simulink model "p1_digital_twin_R2023a"  (R2023a)
settings: Solver=FixedStepDiscrete  StartTime=0.0  StopTime=10  FixedStep=Ts  RelTol=1e-3  EnableMultiTasking=on
values from neighbouring files (symbols this model uses):
  ack = 1    [SteeringController.m]
  cpr_handwheel = 500*4    (= 2000)    [p1_params_new.m]
  cpr_steering = 1000*4    (= 4000)    [p1_params_new.m]
  hal_filter_den = [1 1*(2*pi*Ts)-1]    [SteeringController.m]    (also in p1_params_new.m = DEN_cellarray{1})
  hal_filter_num = [1*(2*pi*Ts)]    [SteeringController.m]    (also in p1_params_new.m = NUM_cellarray{1})
  n_drive = 5.6    [p1_params_new.m]
  n_handwheel = 50    [p1_params_new.m]
  n_steering = 160    [p1_params_new.m]
  sr = 7.5    [SteeringController.m]
  steering_limit = 35    [SteeringController.m]
  Ts = 0.001    [p1_params_new.m]
  wc = 10    [SteeringController.m]    (also in p1_params_new.m = p1params.input.VAccelFc*(2*Ts))
undefined symbols (not defined in the file or in its folder): DiscIntNeverNeededParam, p1params, param
libraries: simulink x7
(part 2 of 4)

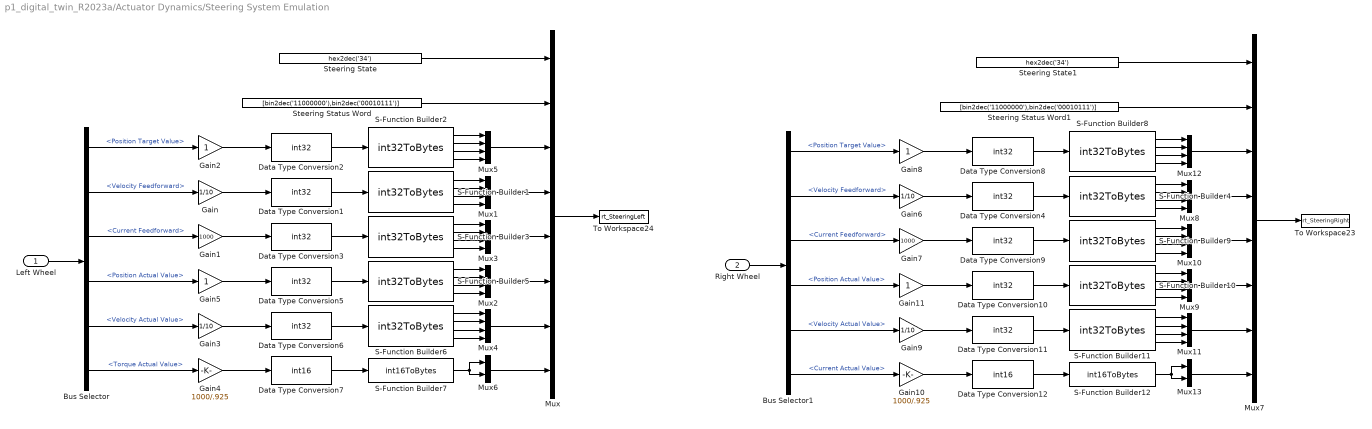
== system p1_digital_twin_R2023a/Actuator Dynamics/Steering System Emulation ==
  Left Wheel : Inport
  Right Wheel : Inport  Port=2
  Bus Selector : BusSelector  OutputSignals=Position Target Value,Velocity Feedforward,Current Feedforward,Position Actual Value,Velocity Actual Value,Torque Actual Value
  Bus Selector1 : BusSelector  OutputSignals=Position Target Value,Velocity Feedforward,Current Feedforward,Position Actual Value,Velocity Actual Value,Current Actual Value
  Data Type Conversion{1..6,8..11} (10 alike) : DataTypeConversion  OutDataTypeStr=int32  RndMeth=Floor
  Data Type Conversion12 : DataTypeConversion  OutDataTypeStr=int16  RndMeth=Floor
  Data Type Conversion7 : DataTypeConversion  OutDataTypeStr=int16  RndMeth=Floor
  Gain{,3,6,9} (4 alike) : Gain  Gain=1/10
  Gain1 : Gain  Gain=1000
  Gain10 : Gain  Gain=1000/.925
  Gain{2,5,8,11} (4 alike) : Gain
  Gain4 : Gain  Gain=1000/.925
  Gain7 : Gain  Gain=1000
  Mux : Mux  Inputs=8
  Mux{1..5,8..12} (10 alike) : Mux
  Mux13 : Mux  Inputs=2
  Mux6 : Mux  Inputs=2
  Mux7 : Mux  Inputs=8
  S-Function Builder1 : S-Function  FunctionName=int32ToBytes  SFunctionModules=int32ToBytes_wrapper.c  SFunctionDeploymentMode=off  EnableBusSupport=off  mask(S-Function Builder){}
      mask help: Simulink:masks:SFunctionBuilder_MD
      mask init:
      | val = [[.9  0.75 0.75 1 1 .9 .9 1]',[1 1 0.75 0.75 .9 .9 1 .9]'];try , sys = get_param(gcb,'SfunBuilderFcnName');if isempty(sys), sys = get_param(gcb,'FunctionName'); end,catch, sys = get_param(gcb,'FunctionName'); end
      settings: CopyFcn=set_param(gcbh,'LinkStatus','none')  OpenFcn=sfunctionwizard(gcbh)
      mask Display:
      | plot(val(:,1),val(:,2))
      | disp(sys)
      | port_label('input',1,'u0')
      | port_label('output',1,'y0')
      | port_label('output',2,'y1')
      | port_label('output',3,'y2')
      | port_label('output',4,'y3')
  S-Function Builder10 : S-Function  FunctionName=int32ToBytes  SFunctionModules=int32ToBytes_wrapper.c  SFunctionDeploymentMode=off  EnableBusSupport=off  mask(S-Function Builder){}
      mask help: Simulink:masks:SFunctionBuilder_MD
      mask init: same as p1_digital_twin_R2023a/Actuator Dynamics/Steering System Emulation/S-Function Builder1
      settings: CopyFcn=set_param(gcbh,'LinkStatus','none')  OpenFcn=sfunctionwizard(gcbh)
      mask Display:
      | plot(val(:,1),val(:,2))
      | disp(sys)
      | port_label('input',1,'u0')
      | port_label('output',1,'y0')
      | port_label('output',2,'y1')
      | port_label('output',3,'y2')
      | port_label('output',4,'y3')
  S-Function Builder11 : S-Function  FunctionName=int32ToBytes  SFunctionModules=int32ToBytes_wrapper.c  SFunctionDeploymentMode=off  EnableBusSupport=off  mask(S-Function Builder){}
      mask help: Simulink:masks:SFunctionBuilder_MD
      mask init: same as p1_digital_twin_R2023a/Actuator Dynamics/Steering System Emulation/S-Function Builder1
      settings: CopyFcn=set_param(gcbh,'LinkStatus','none')  OpenFcn=sfunctionwizard(gcbh)
      mask Display:
      | plot(val(:,1),val(:,2))
      | disp(sys)
      | port_label('input',1,'u0')
      | port_label('output',1,'y0')
      | port_label('output',2,'y1')
      | port_label('output',3,'y2')
      | port_label('output',4,'y3')
  S-Function Builder12 : S-Function  FunctionName=int16ToBytes  SFunctionModules=int16ToBytes_wrapper.c  SFunctionDeploymentMode=off  EnableBusSupport=off  mask(S-Function Builder){}
      mask help: Simulink:masks:SFunctionBuilder_MD
      mask init: same as p1_digital_twin_R2023a/Actuator Dynamics/Steering System Emulation/S-Function Builder1
      settings: CopyFcn=set_param(gcbh,'LinkStatus','none')  OpenFcn=sfunctionwizard(gcbh)
      mask Display:
      | plot(val(:,1),val(:,2))
      | disp(sys)
      | port_label('input',1,'u0')
      | port_label('output',1,'y0')
  S-Function Builder2 : S-Function  FunctionName=int32ToBytes  SFunctionModules=int32ToBytes_wrapper.c  SFunctionDeploymentMode=off  EnableBusSupport=off  mask(S-Function Builder){}
      mask help: Simulink:masks:SFunctionBuilder_MD
      mask init: same as p1_digital_twin_R2023a/Actuator Dynamics/Steering System Emulation/S-Function Builder1
      settings: CopyFcn=set_param(gcbh,'LinkStatus','none')  OpenFcn=sfunctionwizard(gcbh)
      mask Display:
      | plot(val(:,1),val(:,2))
      | disp(sys)
      | port_label('input',1,'u0')
      | port_label('output',1,'y0')
      | port_label('output',2,'y1')
      | port_label('output',3,'y2')
      | port_label('output',4,'y3')
  S-Function Builder3 : S-Function  FunctionName=int32ToBytes  SFunctionModules=int32ToBytes_wrapper.c  SFunctionDeploymentMode=off  EnableBusSupport=off  mask(S-Function Builder){}
      mask help: Simulink:masks:SFunctionBuilder_MD
      mask init: same as p1_digital_twin_R2023a/Actuator Dynamics/Steering System Emulation/S-Function Builder1
      settings: CopyFcn=set_param(gcbh,'LinkStatus','none')  OpenFcn=sfunctionwizard(gcbh)
      mask Display:
      | plot(val(:,1),val(:,2))
      | disp(sys)
      | port_label('input',1,'u0')
      | port_label('output',1,'y0')
      | port_label('output',2,'y1')
      | port_label('output',3,'y2')
      | port_label('output',4,'y3')
  S-Function Builder4 : S-Function  FunctionName=int32ToBytes  SFunctionModules=int32ToBytes_wrapper.c  SFunctionDeploymentMode=off  EnableBusSupport=off  mask(S-Function Builder){}
      mask help: Simulink:masks:SFunctionBuilder_MD
      mask init: same as p1_digital_twin_R2023a/Actuator Dynamics/Steering System Emulation/S-Function Builder1
      settings: CopyFcn=set_param(gcbh,'LinkStatus','none')  OpenFcn=sfunctionwizard(gcbh)
      mask Display:
      | plot(val(:,1),val(:,2))
      | disp(sys)
      | port_label('input',1,'u0')
      | port_label('output',1,'y0')
      | port_label('output',2,'y1')
      | port_label('output',3,'y2')
      | port_label('output',4,'y3')
  S-Function Builder5 : S-Function  FunctionName=int32ToBytes  SFunctionModules=int32ToBytes_wrapper.c  SFunctionDeploymentMode=off  EnableBusSupport=off  mask(S-Function Builder){}
      mask help: Simulink:masks:SFunctionBuilder_MD
      mask init: same as p1_digital_twin_R2023a/Actuator Dynamics/Steering System Emulation/S-Function Builder1
      settings: CopyFcn=set_param(gcbh,'LinkStatus','none')  OpenFcn=sfunctionwizard(gcbh)
      mask Display:
      | plot(val(:,1),val(:,2))
      | disp(sys)
      | port_label('input',1,'u0')
      | port_label('output',1,'y0')
      | port_label('output',2,'y1')
      | port_label('output',3,'y2')
      | port_label('output',4,'y3')
  S-Function Builder6 : S-Function  FunctionName=int32ToBytes  SFunctionModules=int32ToBytes_wrapper.c  SFunctionDeploymentMode=off  EnableBusSupport=off  mask(S-Function Builder){}
      mask help: Simulink:masks:SFunctionBuilder_MD
      mask init: same as p1_digital_twin_R2023a/Actuator Dynamics/Steering System Emulation/S-Function Builder1
      settings: CopyFcn=set_param(gcbh,'LinkStatus','none')  OpenFcn=sfunctionwizard(gcbh)
      mask Display:
      | plot(val(:,1),val(:,2))
      | disp(sys)
      | port_label('input',1,'u0')
      | port_label('output',1,'y0')
      | port_label('output',2,'y1')
      | port_label('output',3,'y2')
      | port_label('output',4,'y3')
  S-Function Builder7 : S-Function  FunctionName=int16ToBytes  SFunctionModules=int16ToBytes_wrapper.c  SFunctionDeploymentMode=off  EnableBusSupport=off  mask(S-Function Builder){}
      mask help: Simulink:masks:SFunctionBuilder_MD
      mask init: same as p1_digital_twin_R2023a/Actuator Dynamics/Steering System Emulation/S-Function Builder1
      settings: CopyFcn=set_param(gcbh,'LinkStatus','none')  OpenFcn=sfunctionwizard(gcbh)
      mask Display:
      | plot(val(:,1),val(:,2))
      | disp(sys)
      | port_label('input',1,'u0')
      | port_label('output',1,'y0')
  S-Function Builder8 : S-Function  FunctionName=int32ToBytes  SFunctionModules=int32ToBytes_wrapper.c  SFunctionDeploymentMode=off  EnableBusSupport=off  mask(S-Function Builder){}
      mask help: Simulink:masks:SFunctionBuilder_MD
      mask init: same as p1_digital_twin_R2023a/Actuator Dynamics/Steering System Emulation/S-Function Builder1
      settings: CopyFcn=set_param(gcbh,'LinkStatus','none')  OpenFcn=sfunctionwizard(gcbh)
      mask Display:
      | plot(val(:,1),val(:,2))
      | disp(sys)
      | port_label('input',1,'u0')
      | port_label('output',1,'y0')
      | port_label('output',2,'y1')
      | port_label('output',3,'y2')
      | port_label('output',4,'y3')
  S-Function Builder9 : S-Function  FunctionName=int32ToBytes  SFunctionModules=int32ToBytes_wrapper.c  SFunctionDeploymentMode=off  EnableBusSupport=off  mask(S-Function Builder){}
      mask help: Simulink:masks:SFunctionBuilder_MD
      mask init: same as p1_digital_twin_R2023a/Actuator Dynamics/Steering System Emulation/S-Function Builder1
      settings: CopyFcn=set_param(gcbh,'LinkStatus','none')  OpenFcn=sfunctionwizard(gcbh)
      mask Display:
      | plot(val(:,1),val(:,2))
      | disp(sys)
      | port_label('input',1,'u0')
      | port_label('output',1,'y0')
      | port_label('output',2,'y1')
      | port_label('output',3,'y2')
      | port_label('output',4,'y3')
  Steering State : Constant  Value=hex2dec('34')  OutDataTypeStr=uint8  SampleTime=-1
  Steering State1 : Constant  Value=hex2dec('34')  OutDataTypeStr=uint8  SampleTime=-1
  Steering Status Word : Constant  Value=[bin2dec('11000000'),bin2dec('00010111')]  OutDataTypeStr=uint8  SampleTime=-1
  Steering Status Word1 : Constant  Value=[bin2dec('11000000'),bin2dec('00010111')]  OutDataTypeStr=uint8  SampleTime=-1
  To Workspace23 : ToWorkspace  VariableName=rt_SteeringRight  SampleTime=-1
  To Workspace24 : ToWorkspace  VariableName=rt_SteeringLeft  SampleTime=-1
  wires:
  Mux/1 -> To Workspace24/1
  Steering State/1 -> Mux/1
  Mux5/1 -> Mux/3
  S-Function Builder2/3 -> Mux5/3
  S-Function Builder2/1 -> Mux5/1
  S-Function Builder2/4 -> Mux5/4
  S-Function Builder2/2 -> Mux5/2
  Steering Status Word/1 -> Mux/2
  S-Function Builder1/4 -> Mux1/4
  S-Function Builder1/1 -> Mux1/1
  S-Function Builder1/2 -> Mux1/2
  S-Function Builder1/3 -> Mux1/3
  Mux1/1 -> Mux/4
  Mux2/1 -> Mux/6
  S-Function Builder3/4 -> Mux3/4
  S-Function Builder3/1 -> Mux3/1
  S-Function Builder3/2 -> Mux3/2
  S-Function Builder3/3 -> Mux3/3
  Mux3/1 -> Mux/5
  S-Function Builder5/3 -> Mux2/3
  S-Function Builder5/1 -> Mux2/1
  S-Function Builder5/2 -> Mux2/2
  S-Function Builder5/4 -> Mux2/4
  Mux4/1 -> Mux/7
  S-Function Builder6/3 -> Mux4/3
  S-Function Builder6/4 -> Mux4/4
  S-Function Builder6/2 -> Mux4/2
  S-Function Builder6/1 -> Mux4/1
  Mux6/1 -> Mux/8
  Data Type Conversion2/1 -> S-Function Builder2/1
  Data Type Conversion1/1 -> S-Function Builder1/1
  Data Type Conversion3/1 -> S-Function Builder3/1
  Data Type Conversion5/1 -> S-Function Builder5/1
  Data Type Conversion6/1 -> S-Function Builder6/1
  Data Type Conversion7/1 -> S-Function Builder7/1
  S-Function Builder7/1 -> Mux6/2, Mux6/1
  Gain2/1 -> Data Type Conversion2/1
  Gain/1 -> Data Type Conversion1/1
  Gain1/1 -> Data Type Conversion3/1
  Gain5/1 -> Data Type Conversion5/1
  Gain3/1 -> Data Type Conversion6/1
  Left Wheel/1 -> Bus Selector/1
  Bus Selector/1 -> Gain2/1  "<Position Target Value>"
  Bus Selector/2 -> Gain/1  "<Velocity Feedforward>"
  Bus Selector/3 -> Gain1/1  "<Current Feedforward>"
  Bus Selector/4 -> Gain5/1  "<Position Actual Value>"
  Bus Selector/5 -> Gain3/1  "<Velocity Actual Value>"
  Bus Selector/6 -> Gain4/1  "<Torque Actual Value>"
  Mux10/1 -> Mux7/5
  Gain9/1 -> Data Type Conversion11/1
  Gain10/1 -> Data Type Conversion12/1
  Right Wheel/1 -> Bus Selector1/1
  S-Function Builder12/1 -> Mux13/2, Mux13/1
  Data Type Conversion11/1 -> S-Function Builder11/1
  Bus Selector1/6 -> Gain10/1  "<Current Actual Value>"
  Mux9/1 -> Mux7/6
  Bus Selector1/3 -> Gain7/1  "<Current Feedforward>"
  Data Type Conversion9/1 -> S-Function Builder9/1
  S-Function Builder9/4 -> Mux10/4
  Gain11/1 -> Data Type Conversion10/1
  S-Function Builder9/3 -> Mux10/3
  S-Function Builder10/4 -> Mux9/4
  Mux12/1 -> Mux7/3
  S-Function Builder11/2 -> Mux11/2
  Data Type Conversion8/1 -> S-Function Builder8/1
  S-Function Builder8/4 -> Mux12/4
  S-Function Builder9/1 -> Mux10/1
  S-Function Builder10/1 -> Mux9/1
  S-Function Builder10/2 -> Mux9/2
  Data Type Conversion10/1 -> S-Function Builder10/1
  Data Type Conversion4/1 -> S-Function Builder4/1
  S-Function Builder4/1 -> Mux8/1
  S-Function Builder8/3 -> Mux12/3
  Mux8/1 -> Mux7/4
  S-Function Builder9/2 -> Mux10/2
  Gain8/1 -> Data Type Conversion8/1
  S-Function Builder8/1 -> Mux12/1
  S-Function Builder8/2 -> Mux12/2
  Steering Status Word1/1 -> Mux7/2
  Steering State1/1 -> Mux7/1
  S-Function Builder11/1 -> Mux11/1
  Gain7/1 -> Data Type Conversion9/1
  S-Function Builder10/3 -> Mux9/3
  Bus Selector1/5 -> Gain9/1  "<Velocity Actual Value>"
  S-Function Builder4/3 -> Mux8/3
  Bus Selector1/1 -> Gain8/1  "<Position Target Value>"
  Bus Selector1/4 -> Gain11/1  "<Position Actual Value>"
  Gain6/1 -> Data Type Conversion4/1
  S-Function Builder4/2 -> Mux8/2
  Bus Selector1/2 -> Gain6/1  "<Velocity Feedforward>"
  S-Function Builder4/4 -> Mux8/4
  Mux11/1 -> Mux7/7
  Mux13/1 -> Mux7/8
  Data Type Conversion12/1 -> S-Function Builder12/1
  S-Function Builder11/4 -> Mux11/4
  S-Function Builder11/3 -> Mux11/3
  Mux7/1 -> To Workspace23/1
  Gain4/1 -> Data Type Conversion7/1

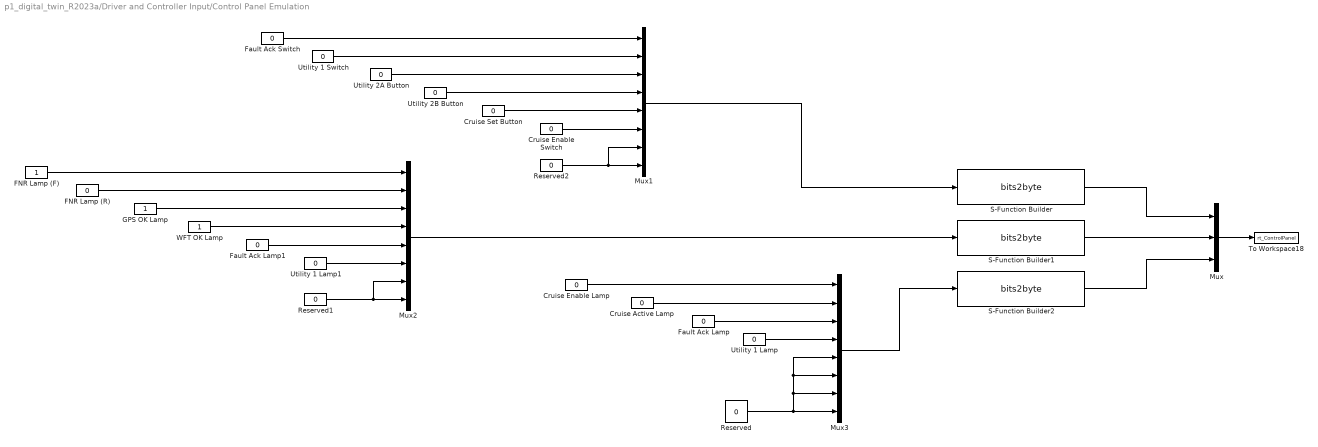
== system p1_digital_twin_R2023a/Driver and Controller Input/Control Panel Emulation ==
  Cruise Active Lamp : Constant  Value=0  OutDataTypeStr=uint8
  Cruise Enable Lamp : Constant  Value=0  OutDataTypeStr=uint8
  Cruise Enable Switch : Constant  Value=0  OutDataTypeStr=uint8
  Cruise Set Button : Constant  Value=0  OutDataTypeStr=uint8
  FNR Lamp (F) : Constant  OutDataTypeStr=uint8
  FNR Lamp (R) : Constant  Value=0  OutDataTypeStr=uint8
  Fault Ack Lamp : Constant  Value=0  OutDataTypeStr=uint8
  Fault Ack Lamp1 : Constant  Value=0  OutDataTypeStr=uint8
  Fault Ack Switch : Constant  Value=0  OutDataTypeStr=uint8  SampleTime=-1
  GPS OK Lamp : Constant  OutDataTypeStr=uint8
  Mux : Mux  Inputs=3
  Mux1 : Mux  Inputs=8
  Mux2 : Mux  Inputs=8
  Mux3 : Mux  Inputs=8
  Reserved : Constant  Value=0  OutDataTypeStr=uint8
  Reserved1 : Constant  Value=0  OutDataTypeStr=uint8
  Reserved2 : Constant  Value=0  OutDataTypeStr=uint8
  S-Function Builder : S-Function  FunctionName=bits2byte  SFunctionModules=bits2byte_wrapper.c  SFunctionDeploymentMode=off  EnableBusSupport=off  mask(S-Function Builder){}
      mask help: Simulink:masks:SFunctionBuilder_MD
      mask init: same as p1_digital_twin_R2023a/Actuator Dynamics/Steering System Emulation/S-Function Builder1
      settings: CopyFcn=set_param(gcbh,'LinkStatus','none')  OpenFcn=sfunctionwizard(gcbh)
      mask Display:
      | plot(val(:,1),val(:,2))
      | disp(sys)
      | port_label('input',1,'u0')
      | port_label('output',1,'y0')
  S-Function Builder1 : S-Function  FunctionName=bits2byte  SFunctionModules=bits2byte_wrapper.c  SFunctionDeploymentMode=off  EnableBusSupport=off  mask(S-Function Builder){}
      mask help: Simulink:masks:SFunctionBuilder_MD
      mask init: same as p1_digital_twin_R2023a/Actuator Dynamics/Steering System Emulation/S-Function Builder1
      settings: CopyFcn=set_param(gcbh,'LinkStatus','none')  OpenFcn=sfunctionwizard(gcbh)
      mask Display:
      | plot(val(:,1),val(:,2))
      | disp(sys)
      | port_label('input',1,'u0')
      | port_label('output',1,'y0')
  S-Function Builder2 : S-Function  FunctionName=bits2byte  SFunctionModules=bits2byte_wrapper.c  SFunctionDeploymentMode=off  EnableBusSupport=off  mask(S-Function Builder){}
      mask help: Simulink:masks:SFunctionBuilder_MD
      mask init: same as p1_digital_twin_R2023a/Actuator Dynamics/Steering System Emulation/S-Function Builder1
      settings: CopyFcn=set_param(gcbh,'LinkStatus','none')  OpenFcn=sfunctionwizard(gcbh)
      mask Display:
      | plot(val(:,1),val(:,2))
      | disp(sys)
      | port_label('input',1,'u0')
      | port_label('output',1,'y0')
  To Workspace18 : ToWorkspace  VariableName=rt_ControlPanel  SampleTime=-1
      settings: Save2DSignal=2-D array (concatenate along first dimension)
  Utility 1 Lamp : Constant  Value=0  OutDataTypeStr=uint8
  Utility 1 Lamp1 : Constant  Value=0  OutDataTypeStr=uint8
  Utility 1 Switch : Constant  Value=0  OutDataTypeStr=uint8
  Utility 2A Button : Constant  Value=0  OutDataTypeStr=uint8
  Utility 2B Button : Constant  Value=0  OutDataTypeStr=uint8
  WFT OK Lamp : Constant  OutDataTypeStr=uint8
  wires:
  Mux/1 -> To Workspace18/1
  S-Function Builder/1 -> Mux/1
  S-Function Builder1/1 -> Mux/2
  S-Function Builder2/1 -> Mux/3
  Mux2/1 -> S-Function Builder1/1
  Mux3/1 -> S-Function Builder2/1
  Reserved/1 -> Mux3/5, Mux3/6, Mux3/7, Mux3/8
  Cruise Enable Lamp/1 -> Mux3/1
  Cruise Active Lamp/1 -> Mux3/2
  Fault Ack Lamp/1 -> Mux3/3
  Utility 1 Lamp/1 -> Mux3/4
  Reserved1/1 -> Mux2/7, Mux2/8
  Utility 1 Lamp1/1 -> Mux2/6
  GPS OK Lamp/1 -> Mux2/3
  WFT OK Lamp/1 -> Mux2/4
  Fault Ack Lamp1/1 -> Mux2/5
  FNR Lamp (F)/1 -> Mux2/1
  FNR Lamp (R)/1 -> Mux2/2
  Cruise Set Button/1 -> Mux1/5
  Utility 2B Button/1 -> Mux1/4
  Cruise Enable Switch/1 -> Mux1/6
  Utility 2A Button/1 -> Mux1/3
  Mux1/1 -> S-Function Builder/1
  Utility 1 Switch/1 -> Mux1/2
  Reserved2/1 -> Mux1/7, Mux1/8
  Fault Ack Switch/1 -> Mux1/1

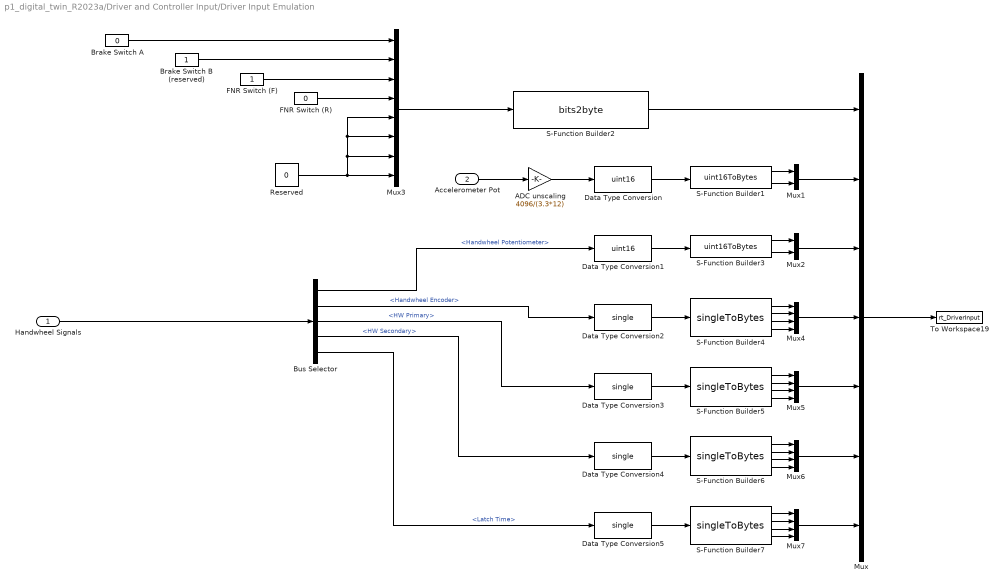
== system p1_digital_twin_R2023a/Driver and Controller Input/Driver Input Emulation ==
  Handwheel Signals : Inport
  Accelerometer Pot : Inport  Port=2
  ADC unscaling : Gain  Gain=4096/(3.3*12)
  Brake Switch A : Constant  Value=0  OutDataTypeStr=uint8  SampleTime=-1
  Brake Switch B (reserved) : Constant  OutDataTypeStr=uint8
  Bus Selector : BusSelector  OutputSignals=Handwheel Potentiometer,Handwheel Encoder,HW Primary,HW Secondary,Latch Time
  Data Type Conversion : DataTypeConversion  OutDataTypeStr=uint16  SaturateOnIntegerOverflow=off  RndMeth=Floor
  Data Type Conversion1 : DataTypeConversion  OutDataTypeStr=uint16  SaturateOnIntegerOverflow=off  RndMeth=Floor
  Data Type Conversion2 : DataTypeConversion  OutDataTypeStr=single  ConvertRealWorld=Stored Integer (SI)  SaturateOnIntegerOverflow=off  RndMeth=Floor
  Data Type Conversion3 : DataTypeConversion  OutDataTypeStr=single  SaturateOnIntegerOverflow=off  RndMeth=Floor
  Data Type Conversion4 : DataTypeConversion  OutDataTypeStr=single  SaturateOnIntegerOverflow=off  RndMeth=Floor
  Data Type Conversion5 : DataTypeConversion  OutDataTypeStr=single  SaturateOnIntegerOverflow=off  RndMeth=Floor
  FNR Switch (F) : Constant  OutDataTypeStr=uint8
  FNR Switch (R) : Constant  Value=0  OutDataTypeStr=uint8
  Mux : Mux  Inputs=7
  Mux1 : Mux  Inputs=2
  Mux2 : Mux  Inputs=2
  Mux3 : Mux  Inputs=8
  Mux{4..7} (4 alike) : Mux
  Reserved : Constant  Value=0  OutDataTypeStr=uint8
  S-Function Builder1 : S-Function  FunctionName=uint16ToBytes  SFunctionModules=uint16ToBytes_wrapper.c  SFunctionDeploymentMode=off  EnableBusSupport=off  mask(S-Function Builder){}
      mask help: Simulink:masks:SFunctionBuilder_MD
      mask init: same as p1_digital_twin_R2023a/Actuator Dynamics/Steering System Emulation/S-Function Builder1
      settings: CopyFcn=set_param(gcbh,'LinkStatus','none')  OpenFcn=sfunctionwizard(gcbh)
      mask Display:
      | plot(val(:,1),val(:,2))
      | disp(sys)
      | port_label('input',1,'u0')
      | port_label('output',1,'y0')
      | port_label('output',2,'y1')
  S-Function Builder2 : S-Function  FunctionName=bits2byte  SFunctionModules=bits2byte_wrapper.c  SFunctionDeploymentMode=off  EnableBusSupport=off  mask(S-Function Builder){}
      mask help: Simulink:masks:SFunctionBuilder_MD
      mask init: same as p1_digital_twin_R2023a/Actuator Dynamics/Steering System Emulation/S-Function Builder1
      settings: CopyFcn=set_param(gcbh,'LinkStatus','none')  OpenFcn=sfunctionwizard(gcbh)
      mask Display:
      | plot(val(:,1),val(:,2))
      | disp(sys)
      | port_label('input',1,'u0')
      | port_label('output',1,'y0')
  S-Function Builder3 : S-Function  FunctionName=uint16ToBytes  SFunctionModules=uint16ToBytes_wrapper.c  SFunctionDeploymentMode=off  EnableBusSupport=off  mask(S-Function Builder){}
      mask help: Simulink:masks:SFunctionBuilder_MD
      mask init: same as p1_digital_twin_R2023a/Actuator Dynamics/Steering System Emulation/S-Function Builder1
      settings: CopyFcn=set_param(gcbh,'LinkStatus','none')  OpenFcn=sfunctionwizard(gcbh)
      mask Display:
      | plot(val(:,1),val(:,2))
      | disp(sys)
      | port_label('input',1,'u0')
      | port_label('output',1,'y0')
      | port_label('output',2,'y1')
  S-Function Builder4 : S-Function  FunctionName=singleToBytes  SFunctionModules=singleToBytes_wrapper.c  SFunctionDeploymentMode=off  EnableBusSupport=off  mask(S-Function Builder){}
      mask help: Simulink:masks:SFunctionBuilder_MD
      mask init: same as p1_digital_twin_R2023a/Actuator Dynamics/Steering System Emulation/S-Function Builder1
      settings: CopyFcn=set_param(gcbh,'LinkStatus','none')  OpenFcn=sfunctionwizard(gcbh)
      mask Display:
      | plot(val(:,1),val(:,2))
      | disp(sys)
      | port_label('input',1,'u0')
      | port_label('output',1,'y0')
      | port_label('output',2,'y1')
      | port_label('output',3,'y2')
      | port_label('output',4,'y3')
  S-Function Builder5 : S-Function  FunctionName=singleToBytes  SFunctionModules=singleToBytes_wrapper.c  SFunctionDeploymentMode=off  EnableBusSupport=off  mask(S-Function Builder){}
      mask help: Simulink:masks:SFunctionBuilder_MD
      mask init: same as p1_digital_twin_R2023a/Actuator Dynamics/Steering System Emulation/S-Function Builder1
      settings: CopyFcn=set_param(gcbh,'LinkStatus','none')  OpenFcn=sfunctionwizard(gcbh)
      mask Display:
      | plot(val(:,1),val(:,2))
      | disp(sys)
      | port_label('input',1,'u0')
      | port_label('output',1,'y0')
      | port_label('output',2,'y1')
      | port_label('output',3,'y2')
      | port_label('output',4,'y3')
  S-Function Builder6 : S-Function  FunctionName=singleToBytes  SFunctionModules=singleToBytes_wrapper.c  SFunctionDeploymentMode=off  EnableBusSupport=off  mask(S-Function Builder){}
      mask help: Simulink:masks:SFunctionBuilder_MD
      mask init: same as p1_digital_twin_R2023a/Actuator Dynamics/Steering System Emulation/S-Function Builder1
      settings: CopyFcn=set_param(gcbh,'LinkStatus','none')  OpenFcn=sfunctionwizard(gcbh)
      mask Display:
      | plot(val(:,1),val(:,2))
      | disp(sys)
      | port_label('input',1,'u0')
      | port_label('output',1,'y0')
      | port_label('output',2,'y1')
  S-Function Builder7 : S-Function  FunctionName=singleToBytes  SFunctionModules=singleToBytes_wrapper.c  SFunctionDeploymentMode=off  EnableBusSupport=off  mask(S-Function Builder){}
      mask help: Simulink:masks:SFunctionBuilder_MD
      mask init: same as p1_digital_twin_R2023a/Actuator Dynamics/Steering System Emulation/S-Function Builder1
      settings: CopyFcn=set_param(gcbh,'LinkStatus','none')  OpenFcn=sfunctionwizard(gcbh)
      mask Display:
      | plot(val(:,1),val(:,2))
      | disp(sys)
      | port_label('input',1,'u0')
      | port_label('output',1,'y0')
      | port_label('output',2,'y1')
  To Workspace19 : ToWorkspace  VariableName=rt_DriverInput  SampleTime=-1
      settings: Save2DSignal=2-D array (concatenate along first dimension)
  wires:
  FNR Switch (R)/1 -> Mux3/4
  Brake Switch A/1 -> Mux3/1
  Brake Switch B (reserved)/1 -> Mux3/2
  Mux3/1 -> S-Function Builder2/1
  FNR Switch (F)/1 -> Mux3/3
  Reserved/1 -> Mux3/5, Mux3/6, Mux3/7, Mux3/8
  Mux/1 -> To Workspace19/1
  S-Function Builder2/1 -> Mux/1
  S-Function Builder1/1 -> Mux1/1
  S-Function Builder1/2 -> Mux1/2
  Mux1/1 -> Mux/2
  Accelerometer Pot/1 -> ADC unscaling/1
  ADC unscaling/1 -> Data Type Conversion/1
  Data Type Conversion/1 -> S-Function Builder1/1
  Mux2/1 -> Mux/3
  Handwheel Signals/1 -> Bus Selector/1
  S-Function Builder3/2 -> Mux2/2
  Data Type Conversion1/1 -> S-Function Builder3/1
  S-Function Builder3/1 -> Mux2/1
  Data Type Conversion2/1 -> S-Function Builder4/1
  S-Function Builder4/1 -> Mux4/1
  Data Type Conversion3/1 -> S-Function Builder5/1
  Data Type Conversion4/1 -> S-Function Builder6/1
  Data Type Conversion5/1 -> S-Function Builder7/1
  Bus Selector/1 -> Data Type Conversion1/1  "<Handwheel Potentiometer>"
  Bus Selector/2 -> Data Type Conversion2/1  "<Handwheel Encoder>"
  Bus Selector/3 -> Data Type Conversion3/1  "<HW Primary>"
  Bus Selector/5 -> Data Type Conversion5/1  "<Latch Time>"
  Bus Selector/4 -> Data Type Conversion4/1  "<HW Secondary>"
  S-Function Builder4/4 -> Mux4/4
  S-Function Builder4/2 -> Mux4/2
  S-Function Builder4/3 -> Mux4/3
  Mux5/1 -> Mux/5
  S-Function Builder5/1 -> Mux5/1
  S-Function Builder5/4 -> Mux5/4
  S-Function Builder5/3 -> Mux5/3
  S-Function Builder5/2 -> Mux5/2
  Mux6/1 -> Mux/6
  S-Function Builder6/1 -> Mux6/1
  S-Function Builder6/2 -> Mux6/2
  S-Function Builder6/4 -> Mux6/4
  S-Function Builder6/3 -> Mux6/3
  S-Function Builder7/1 -> Mux7/1
  S-Function Builder7/4 -> Mux7/4
  S-Function Builder7/2 -> Mux7/2
  S-Function Builder7/3 -> Mux7/3
  Mux7/1 -> Mux/7
  Mux4/1 -> Mux/4

== system p1_digital_twin_R2023a/Driver and Controller Input/Steering Controller ==
  Driver Input : Inport
  Steering Addition : Inport  Port=2
  Ackermann Correction : Subsystem
  Add : Sum
  Bus Selector1 : BusSelector  OutputSignals=HW Primary
  Bus Selector4 : BusSelector  OutputSignals=Utility 1
  D2R : Gain  Gain=pi/180  SaturateOnIntegerOverflow=on  OutDataTypeStr=Inherit: Same as input  ParamDataTypeStr=Inherit: Same as input
  Data Store Read : DataStoreRead  DataStoreName=Toe_Offset  IndexOptions=Index vector (dialog)  Indices=1  OutputSizes=1
  HAL-9000 : Subsystem  mask{enabled=off, maneuver=Chirp, amplitude=5, delay=0, duration=20, startfreq=.5, endfreq=5}
      mask prompts: enabled "Enable HAL-9000 Automated Steering Maneuver System"; maneuver "Steering manuever"; amplitude "Amplitude (deg)"; delay "Delay (sec)"; duration "Duration (sec)"; startfreq "Initial frequency (Hz)"; endfreq "Final frequency (Hz)"
      mask init:
      | switch(maneuver)
      | 	case 'Step'
      | 		maneuver=1;
      | 	case 'Ramp'
      | 		maneuver=2;
      | 	case 'Chirp'
      | 		maneuver=3;
      | 	case 'Double-step'
      | 		maneuver=4;
      | 	case 'Double chirp'
      | 		maneuver=5;
      | end
      | switch(enabled)
      | 	case 'on'
      | 		enabled=1;
      | 	case 'off'
      | 		enabled=0;
      | end
      mask Callback enabled:
      | if(strcmp(get_param(gcb,'enabled'),'off'))
      | 	set_param(gcb,'MaskEnables',{'on','off','off','off','off','off','off'});
      | else
      | 	set_param(gcb,'MaskEnables',{'on','on','on','on','on','on','on'});
      | end
      mask TypeOptions maneuver: Step | Ramp | Chirp | Double step | Double chirp
      mask Callback maneuver:
      | switch(get_param(gcb,'maneuver'))
      | 	case 'Step'
      | 		set_param(gcb,'MaskVisibilities',{'on','on','on','on','off','off','off'});
      | 	case 'Double step'
      | 		set_param(gcb,'MaskVisibilities',{'on','on','on','on','on','off','off'});
      | 	case 'Ramp'
      | 		set_param(gcb,'MaskVisibilities',{'on','on','on','on','on','off','off'});
      | 	case 'Chirp'
      | 		set_param(gcb,'MaskVisibilities',{'on','on','on','on','on','on','on'});
      | 	case 'Double chirp'
      | 		set_param(gcb,'MaskVisibilities',{'on','on','on','on','on','on','on'});
      | end
  Heavy Filter : DiscreteFilter  Numerator=hal_filter_num  Denominator=hal_filter_den  SampleTime=Ts
  Input Selector : Constant  Value=2
  Multiport Switch : MultiPortSwitch  SaturateOnIntegerOverflow=off  InputSameDT=off
  Mux1 : Mux  Inputs=2
  Nominal Filter : DiscreteFilter  Numerator=[wc*2*pi*Ts]  Denominator=[1 wc*2*pi*Ts-1]  SampleTime=Ts
  Software Steering Limit : Saturate  UpperLimit=steering_limit*sr*pi/180  LowerLimit=-steering_limit*sr*pi/180
  Software Steering Limit1 : Saturate  UpperLimit=steering_limit*pi/180  LowerLimit=-steering_limit*pi/180
  Steering Ratio1 : Gain  Gain=sr  SaturateOnIntegerOverflow=on  OutDataTypeStr=Inherit: Same as input  ParamDataTypeStr=Inherit: Same as input
  Steering Ratio : Gain  Gain=1/sr  SaturateOnIntegerOverflow=on  OutDataTypeStr=Inherit: Same as input  ParamDataTypeStr=Inherit: Same as input
  Subtract : Sum  Inputs=-+
  Sum : Sum  Inputs=++|
  Sum1 : Sum  Inputs=+++
  Switch : Switch  Criteria=u2 ~= 0  Threshold=0.5  SaturateOnIntegerOverflow=off  InputSameDT=off
  To Workspace : ToWorkspace  VariableName=SteerAngle  SampleTime=-1
  Steering Angle Commands : Outport
  wires:
  Data Store Read/1 -> D2R/1
  D2R/1 -> Subtract/1, Add/1
  Mux1/1 -> To Workspace/1, Steering Angle Commands/1
  Sum1/1 -> Switch/1
  Switch/1 -> Multiport Switch/4
  Input Selector/1 -> Multiport Switch/1
  HAL-9000/1(Offset) -> Sum1/3
  Heavy Filter/1 -> Sum1/2
  Sum/1 -> Multiport Switch/3
  Nominal Filter/1 -> Switch/3, Multiport Switch/2, Software Steering Limit/1
  Steering Ratio1/1 -> Sum1/1, Sum/2
  Steering Addition/1 -> Steering Ratio1/1
  Bus Selector4/1 -> Switch/2, HAL-9000/1(Trigger)  "<Utility 1>"
  Multiport Switch/1 -> Steering Ratio/1
  Software Steering Limit/1 -> Sum/1
  Software Steering Limit1/1 -> Ackermann Correction/1(Ackermann Angle)
  Steering Ratio/1 -> Software Steering Limit1/1
  Ackermann Correction/1(L Steer Angle) -> Subtract/2
  Ackermann Correction/2(R Steer Angle) -> Add/2
  Subtract/1 -> Mux1/1
  Add/1 -> Mux1/2
  Bus Selector1/1 -> Heavy Filter/1, Nominal Filter/1  "<HW Primary>"
  Driver Input/1 -> Bus Selector4/1, Bus Selector1/1

== system p1_digital_twin_R2023a/Vehicle Chassis Dynamics/Calculate Normals ==
  Lateral Accel : Inport  PortDimensions=1
  Add1 : Sum  Inputs=+-
  Bus Selector1 : BusSelector  OutputSignals=m,h_cg,d
  Bus Selector2 : BusSelector  OutputSignals=b,L,a
  Divide : Product  Inputs=*/
  Divide1 : Product  Inputs=/*
  Mux1 : Mux  Inputs=2
  Mux2 : Mux  Inputs=2
  Mux3 : Mux  Inputs=2
  Product : Product  RndMeth=Zero
  Product1 : Product  RndMeth=Zero
  Product2 : Product  Inputs=/**  RndMeth=Zero
  Product3 : Product  Inputs=**/*  RndMeth=Zero
  Subtract1 : Sum
  constant : Constant  Value=2
  g : Constant  Value=9.81
  Normal Forces : Outport  VectorParamsAs1DForOutWhenUnconnected=off
  wires:
  [Vehicle] -> Bus Selector1/1
  Mux2/1 -> Normal Forces/1
  Bus Selector1/1 -> Product3/1, Product2/3  "<m>"
  Bus Selector1/2 -> Product3/2  "<h_cg>"
  Bus Selector1/3 -> Product3/3  "<d>"
  Lateral Accel/1 -> Product3/4
  Product3/1 -> Subtract1/2, Add1/2
  g/1 -> Product2/2
  constant/1 -> Product2/1
  Product2/1 -> Add1/1, Subtract1/1
  [Vehicle] -> Bus Selector2/1
  Bus Selector2/2 -> Divide/2, Divide1/1  "<L>"
  Divide1/1 -> Product1/1
  Divide/1 -> Product/2
  Bus Selector2/1 -> Divide/1  "<b>"
  Bus Selector2/3 -> Divide1/2  "<a>"
  Add1/1 -> Mux1/1, Mux3/1
  Subtract1/1 -> Mux3/2, Mux1/2
  Product1/1 -> Mux2/2
  Product/1 -> Mux2/1
  Mux1/1 -> Product/1
  Mux3/1 -> Product1/2

== system p1_digital_twin_R2023a/Vehicle Chassis Dynamics/Calculate Slips ==
  Yaw Rate : Inport
  Vy : Inport  Port=2
  Vx : Inport  Port=3
  delta : Inport  Port=4
  Add : Sum
  Bus Selector1 : BusSelector  OutputSignals=a,b
  Divide : Product  Inputs=*/
  Divide1 : Product  Inputs=/*
  Mux : Mux
  Product : Product  RndMeth=Zero
  Product1 : Product  RndMeth=Zero
  Selector : Selector  InputPortWidth=4  IndexOptions=Index vector (dialog)  Indices=[1]  OutputSizes=1
  Selector1 : Selector  InputPortWidth=4  IndexOptions=Index vector (dialog)  Indices=[2]  OutputSizes=1
  Subtract : Sum  Inputs=-+
  Subtract1 : Sum  Inputs=-+
  Subtract2 : Sum  Inputs=-+
  Vy1 : InportShadow  Port=2
  Slip Angles : Outport  VectorParamsAs1DForOutWhenUnconnected=off
  wires:
  [Vehicle] -> Bus Selector1/1
  Yaw Rate/1 -> Product1/2, Product/1
  Bus Selector1/1 -> Product1/1  "<a>"
  Bus Selector1/2 -> Product/2  "<b>"
  Product/1 -> Subtract/1
  Vy1/1 -> Subtract/2
  Mux/1 -> Slip Angles/1
  Product1/1 -> Add/2
  Vx/1 -> Divide/2, Divide1/1
  Add/1 -> Divide/1
  Vy/1 -> Add/1
  Subtract/1 -> Divide1/2
  Divide/1 -> Subtract2/2, Subtract1/2
  Divide1/1 -> Mux/4, Mux/3
  Selector1/1 -> Subtract1/1
  Selector/1 -> Subtract2/1
  delta/1 -> Selector1/1, Selector/1
  Subtract2/1 -> Mux/1
  Subtract1/1 -> Mux/2

== system p1_digital_twin_R2023a/Vehicle Chassis Dynamics/Chassis Model ==
  r : Inport
  Fy : Inport  Port=2
  Ux : Inport  Port=3
  Bus Selector1 : BusSelector  OutputSignals=Izz,a
  Bus Selector2 : BusSelector  OutputSignals=b
  Bus Selector3 : BusSelector  OutputSignals=m
  Divide : Product  Inputs=/*
  Divide1 : Product  Inputs=*/
  Product : Product  RndMeth=Zero
  Product1 : Product  RndMeth=Zero
  Product2 : Product  RndMeth=Zero
  Selector : Selector  InputPortWidth=4  IndexOptions=Index vector (dialog)  Indices=[1 2]  OutputSizes=1
  Selector1 : Selector  InputPortWidth=4  IndexOptions=Index vector (dialog)  Indices=[3 4]  OutputSizes=1
  Subtract : Sum  Inputs=+-
  Subtract1 : Sum  Inputs=+-
  Sum of Elements : Sum  Inputs=+
  Sum of Elements1 : Sum  Inputs=+
  Sum of Elements2 : Sum  Inputs=+
  rdot : Outport  VectorParamsAs1DForOutWhenUnconnected=off
  Vydot : Outport  Port=2  VectorParamsAs1DForOutWhenUnconnected=off
  ay : Outport  Port=3  VectorParamsAs1DForOutWhenUnconnected=off
  wires:
  Fy/1 -> Selector/1, Selector1/1, Sum of Elements2/1
  Divide/1 -> rdot/1
  [Vehicle] -> Bus Selector1/1
  Selector/1 -> Sum of Elements/1
  Selector1/1 -> Sum of Elements1/1
  Sum of Elements/1 -> Product/2
  Bus Selector1/2 -> Product/1  "<a>"
  [Vehicle] -> Bus Selector2/1
  Sum of Elements1/1 -> Product1/1
  Bus Selector2/1 -> Product1/2  "<b>"
  Bus Selector1/1 -> Divide/1  "<Izz>"
  Product/1 -> Subtract/1
  Product1/1 -> Subtract/2
  Subtract/1 -> Divide/2
  [Vehicle] -> Bus Selector3/1
  Sum of Elements2/1 -> Divide1/1
  Bus Selector3/1 -> Divide1/2  "<m>"
  Divide1/1 -> Subtract1/1, ay/1
  Subtract1/1 -> Vydot/1
  Ux/1 -> Product2/2
  r/1 -> Product2/1
  Product2/1 -> Subtract1/2

== system p1_digital_twin_R2023a/Vehicle Chassis Dynamics/Drivetrain Dynamics ==
  note: Need to figure out how to handle regen properly
      | and power limits for continous operation.
  Motor Torque Requests : Inport
  Wheel Speeds : Inport  Port=2
  1-D Lookup Table : Lookup_n-D  NumberOfTableDimensions=1  BreakpointsForDimension1=[0 1000 2000 3000 4000 5000 6000 7000 8000 9000 10000]  BeginIndexSearchUsingPreviousIndexResult=on  Table=[350 350 330 330 300 290 250 220 195 175 155]  ExtrapMethod=Clip  UseLastTableValue=on  InternalRulePriority=Speed  RndMeth=Simplest
  Gain : Gain  Gain=1/n_drive
  Gain1 : Gain  Gain=-1
  Gain2 : Gain  Gain=n_drive
  Saturation Dynamic : simulink/Discontinuities/Saturation Dynamic  OutMin=[]  OutMax=[]  OutDataTypeStr=Inherit: Same as second input  OutDataType=fixdt(1, 16)  OutScaling=2^-10  DoSatur=off
  Wheel Torques : Outport
  wires:
  Wheel Speeds/1 -> Gain/1
  Motor Torque Requests/1 -> Saturation Dynamic/2
  1-D Lookup Table/1 -> Gain1/1, Saturation Dynamic/1
  Gain1/1 -> Saturation Dynamic/3
  Gain/1 -> 1-D Lookup Table/1
  Saturation Dynamic/1 -> Gain2/1
  Gain2/1 -> Wheel Torques/1

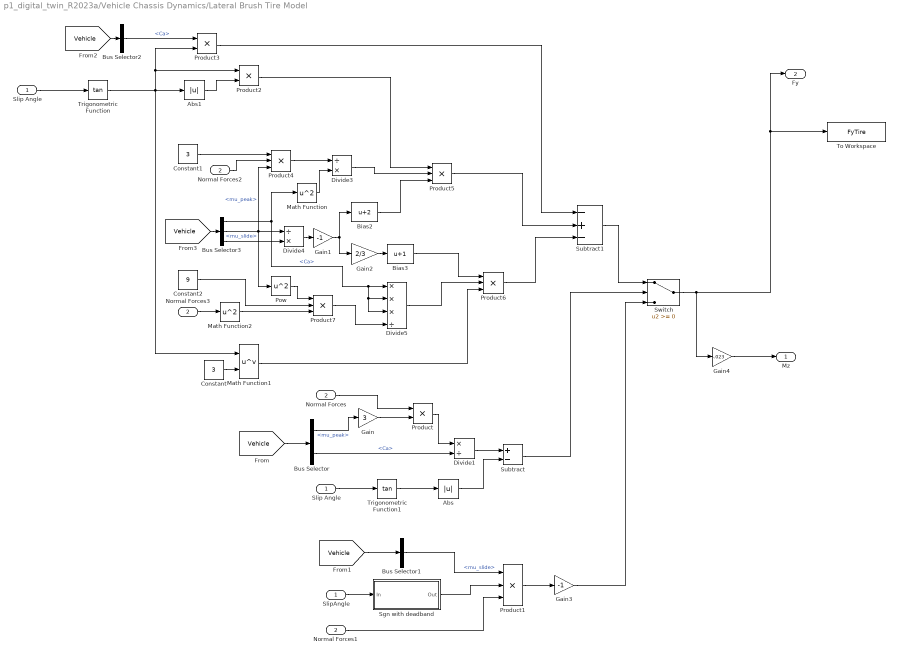
== system p1_digital_twin_R2023a/Vehicle Chassis Dynamics/Lateral Brush Tire Model ==
  SlipAngle : Inport
  Normal Forces : Inport  Port=2
  Abs : Abs  ZeroCross=off  SaturateOnIntegerOverflow=off
  Abs1 : Abs  ZeroCross=off  SaturateOnIntegerOverflow=off
  Bias2 : Bias  Bias=2  SaturateOnIntegerOverflow=off
  Bias3 : Bias  Bias=1  SaturateOnIntegerOverflow=off
  Bus Selector : BusSelector  OutputSignals=mu_peak,Ca
  Bus Selector1 : BusSelector  OutputSignals=mu_slide
  Bus Selector2 : BusSelector  OutputSignals=Ca
  Bus Selector3 : BusSelector  OutputSignals=Ca,mu_peak,mu_slide
  Constant : Constant  Value=3
  Constant1 : Constant  Value=3
  Constant2 : Constant  Value=9
  Divide1 : Product  Inputs=*/
  Divide3 : Product  Inputs=/*
  Divide4 : Product  Inputs=/*
  Divide5 : Product  Inputs=***/
  Gain : Gain  Gain=3
  Gain1 : Gain  Gain=-1
  Gain2 : Gain  Gain=2/3
  Gain3 : Gain  Gain=-1
  Gain4 : Gain  Gain=-.023
  Math Function : Math  Operator=square  SignedPower=on
  Math Function1 : Math  Operator=pow  SignedPower=on
  Math Function2 : Math  Operator=square  SignedPower=on
  Normal Forces1 : InportShadow  Port=2
  Normal Forces2 : InportShadow  Port=2
  Normal Forces3 : InportShadow  Port=2
  Pow : Math  Operator=square  SignedPower=on
  Product : Product  RndMeth=Zero
  Product{1,4..7} (5 alike) : Product  Inputs=3  RndMeth=Zero
  Product2 : Product  RndMeth=Zero
  Product3 : Product  RndMeth=Zero
  Sgn with deadband : Subsystem  mask{lower_dz=-0.01, upper_dz=0.01}
      mask prompts: lower_dz "Lower Dead Zone Boundary"; upper_dz "Upper Dead Zone Boundary"
  Slip Angle : InportShadow
  "Slip Angle " : InportShadow
  Subtract : Sum  Inputs=+-
  Subtract1 : Sum  Inputs=-+-
  Switch : Switch  SaturateOnIntegerOverflow=off  InputSameDT=off
  To Workspace : ToWorkspace  VariableName=FyTire  SampleTime=-1
  Trigonometric Function : Trigonometry  Operator=tan
  Trigonometric Function1 : Trigonometry  Operator=tan
  Mz : Outport
  Fy : Outport  Port=2  VectorParamsAs1DForOutWhenUnconnected=off
  wires:
  [Vehicle] -> Bus Selector/1
  Trigonometric Function1/1 -> Abs/1
  Abs/1 -> Subtract/2
  Bus Selector/2 -> Divide1/2  "<Ca>"
  Divide1/1 -> Subtract/1
  Normal Forces/1 -> Product/1
  Product/1 -> Divide1/1
  Bus Selector/1 -> Gain/1  "<mu_peak>"
  Gain/1 -> Product/2
  Switch/1 -> To Workspace/1, Fy/1, Gain4/1
  SlipAngle/1 -> Sgn with deadband/1(In)
  [Vehicle] -> Bus Selector1/1
  Bus Selector1/1 -> Product1/1  "<mu_slide>"
  Sgn with deadband/1(Out) -> Product1/2
  Normal Forces1/1 -> Product1/3
  [Vehicle] -> Bus Selector2/1
  Trigonometric Function/1 -> Abs1/1, Math Function1/1, Product2/1, Product3/2
  Slip Angle/1 -> Trigonometric Function/1
  Constant/1 -> Math Function1/2
  Abs1/1 -> Product2/2
  Bus Selector2/1 -> Product3/1  "<Ca>"
  Product3/1 -> Subtract1/1
  [Vehicle] -> Bus Selector3/1
  Constant1/1 -> Product4/1
  Normal Forces2/1 -> Product4/2
  Bus Selector3/2 -> Divide4/1, Product4/3, Pow/1  "<mu_peak>"
  Bus Selector3/1 -> Math Function/1, Divide5/1, Divide5/2, Divide5/3  "<Ca>"
  Product4/1 -> Divide3/1
  Math Function/1 -> Divide3/2
  Bus Selector3/3 -> Divide4/2  "<mu_slide>"
  Divide4/1 -> Gain1/1
  Gain1/1 -> Bias2/1, Gain2/1
  Gain2/1 -> Bias3/1
  Bias2/1 -> Product5/3
  Divide3/1 -> Product5/2
  Product2/1 -> Product5/1
  Product5/1 -> Subtract1/2
  Math Function1/1 -> Product6/3
  Bias3/1 -> Product6/1
  Normal Forces3/1 -> Math Function2/1
  Constant2/1 -> Product7/2
  Math Function2/1 -> Product7/3
  Pow/1 -> Product7/1
  Divide5/1 -> Product6/2
  Product6/1 -> Subtract1/3
  Subtract1/1 -> Switch/1
  Product7/1 -> Divide5/4
  Product1/1 -> Gain3/1
  Subtract/1 -> Switch/2
  "Slip Angle "/1 -> Trigonometric Function1/1
  Gain3/1 -> Switch/3
  Gain4/1 -> Mz/1

== system p1_digital_twin_R2023a/Vehicle Chassis Dynamics/Rolling Resistance ==
  In1 : Inport
  In3 : Inport  Port=2
  In2 : Inport  Port=3
  Add1 : Sum  Inputs=+++
  Add2 : Sum
  Bus Selector : BusSelector  OutputSignals=Ca
  Constant2 : Constant  Value=1/0.2921
  Constant3 : Constant  Value=sin((pi/180)*3.5)
  Gain : Gain  Gain=0.013
  Gain3 : Gain  Gain=-1
  Gain4 : Gain  Gain=cos((pi/180)*3.5)
  Product15 : Product  Inputs=3
  Product3 : Product
  Square : Math  Operator=square
  Output : Outport
  wires:
  Square/1 -> Gain3/1
  Gain3/1 -> Product3/1
  Bus Selector/1 -> Product3/2  "<Ca>"
  In2/1 -> Product15/1
  Constant3/1 -> Product15/3
  Gain4/1 -> Add2/1
  Gain/1 -> Gain4/1, Add1/1
  Product3/1 -> Add1/2
  [Vehicle] -> Bus Selector/1
  Constant2/1 -> Product15/2
  Product15/1 -> Add2/2
  Add2/1 -> Add1/3
  In3/1 -> Gain/1
  In1/1 -> Square/1
  Add1/1 -> Output/1

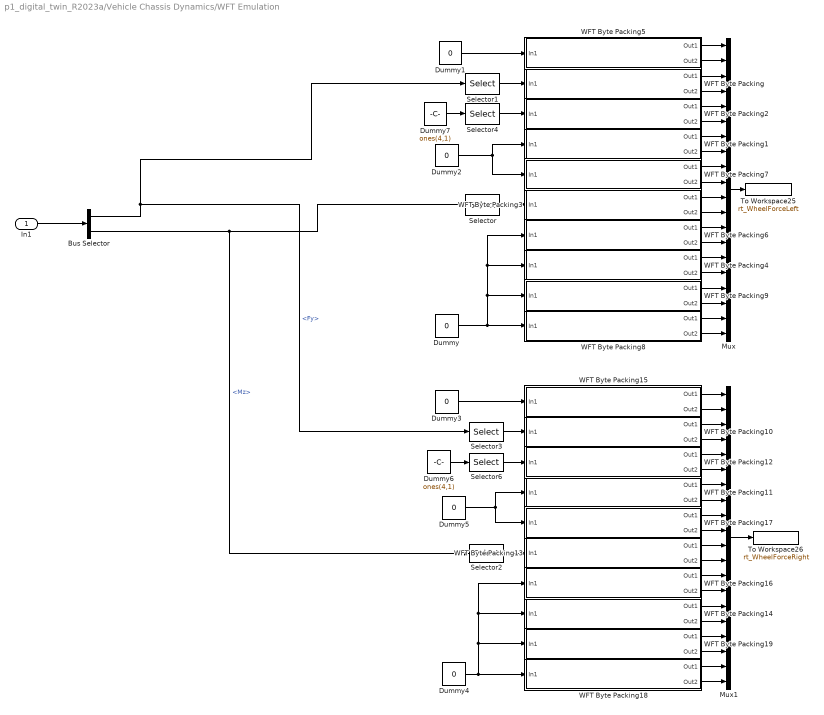
== system p1_digital_twin_R2023a/Vehicle Chassis Dynamics/WFT Emulation ==
  In1 : Inport
  Bus Selector : BusSelector  OutputSignals=Fy,Mz
  Dummy{,1..5} (6 alike) : Constant  Value=0
  Dummy6 : Constant  Value=ones(4,1)
  Dummy7 : Constant  Value=ones(4,1)
  Mux : Mux  Inputs=20
  Mux1 : Mux  Inputs=20
  Selector : Selector  InputPortWidth=4  IndexOptions=Index vector (dialog)  Indices=1  OutputSizes=1
  Selector1 : Selector  InputPortWidth=4  IndexOptions=Index vector (dialog)  Indices=1  OutputSizes=1
  Selector2 : Selector  InputPortWidth=4  IndexOptions=Index vector (dialog)  Indices=2  OutputSizes=1
  Selector3 : Selector  InputPortWidth=4  IndexOptions=Index vector (dialog)  Indices=2  OutputSizes=1
  Selector4 : Selector  InputPortWidth=4  IndexOptions=Index vector (dialog)  Indices=1  OutputSizes=1
  Selector6 : Selector  InputPortWidth=4  IndexOptions=Index vector (dialog)  Indices=2  OutputSizes=1
  To Workspace25 : ToWorkspace  VariableName=rt_WheelForceLeft  SampleTime=-1
      settings: Save2DSignal=2-D array (concatenate along first dimension)
  To Workspace26 : ToWorkspace  VariableName=rt_WheelForceRight  SampleTime=-1
      settings: Save2DSignal=2-D array (concatenate along first dimension)
  WFT Byte Packing : Subsystem
  WFT Byte Packing1 : Subsystem
  WFT Byte Packing10 : Subsystem
  WFT Byte Packing11 : Subsystem
  WFT Byte Packing12 : Subsystem
  WFT Byte Packing13 : Subsystem
  WFT Byte Packing14 : Subsystem
  WFT Byte Packing15 : Subsystem
  WFT Byte Packing16 : Subsystem
  WFT Byte Packing17 : Subsystem
  WFT Byte Packing18 : Subsystem
  WFT Byte Packing19 : Subsystem
  WFT Byte Packing2 : Subsystem
  WFT Byte Packing3 : Subsystem
  WFT Byte Packing4 : Subsystem
  WFT Byte Packing5 : Subsystem
  WFT Byte Packing6 : Subsystem
  WFT Byte Packing7 : Subsystem
  WFT Byte Packing8 : Subsystem
  WFT Byte Packing9 : Subsystem
  wires:
  WFT Byte Packing/2(Out2) -> Mux/4
  WFT Byte Packing12/2(Out2) -> Mux1/6
  Selector/1 -> WFT Byte Packing3/1(In1)
  WFT Byte Packing5/2(Out2) -> Mux/2
  WFT Byte Packing2/2(Out2) -> Mux/6
  WFT Byte Packing1/1(Out1) -> Mux/7
  WFT Byte Packing9/2(Out2) -> Mux/18
  WFT Byte Packing6/2(Out2) -> Mux/14
  WFT Byte Packing8/1(Out1) -> Mux/19
  WFT Byte Packing6/1(Out1) -> Mux/13
  Selector1/1 -> WFT Byte Packing/1(In1)
  WFT Byte Packing2/1(Out1) -> Mux/5
  WFT Byte Packing15/1(Out1) -> Mux1/1
  WFT Byte Packing1/2(Out2) -> Mux/8
  WFT Byte Packing9/1(Out1) -> Mux/17
  Mux/1 -> To Workspace25/1
  WFT Byte Packing14/2(Out2) -> Mux1/16
  WFT Byte Packing18/1(Out1) -> Mux1/19
  WFT Byte Packing19/2(Out2) -> Mux1/18
  Mux1/1 -> To Workspace26/1
  WFT Byte Packing3/1(Out1) -> Mux/11
  WFT Byte Packing7/1(Out1) -> Mux/9
  WFT Byte Packing11/2(Out2) -> Mux1/8
  WFT Byte Packing8/2(Out2) -> Mux/20
  WFT Byte Packing4/1(Out1) -> Mux/15
  Dummy1/1 -> WFT Byte Packing5/1(In1)
  Selector2/1 -> WFT Byte Packing13/1(In1)
  WFT Byte Packing16/2(Out2) -> Mux1/14
  WFT Byte Packing13/1(Out1) -> Mux1/11
  WFT Byte Packing19/1(Out1) -> Mux1/17
  WFT Byte Packing18/2(Out2) -> Mux1/20
  WFT Byte Packing13/2(Out2) -> Mux1/12
  WFT Byte Packing14/1(Out1) -> Mux1/15
  WFT Byte Packing5/1(Out1) -> Mux/1
  Dummy3/1 -> WFT Byte Packing15/1(In1)
  WFT Byte Packing3/2(Out2) -> Mux/12
  WFT Byte Packing17/2(Out2) -> Mux1/10
  WFT Byte Packing/1(Out1) -> Mux/3
  WFT Byte Packing11/1(Out1) -> Mux1/7
  WFT Byte Packing12/1(Out1) -> Mux1/5
  Selector6/1 -> WFT Byte Packing12/1(In1)
  WFT Byte Packing10/2(Out2) -> Mux1/4
  WFT Byte Packing10/1(Out1) -> Mux1/3
  WFT Byte Packing16/1(Out1) -> Mux1/13
  WFT Byte Packing17/1(Out1) -> Mux1/9
  Selector4/1 -> WFT Byte Packing2/1(In1)
  Dummy7/1 -> Selector4/1
  WFT Byte Packing7/2(Out2) -> Mux/10
  WFT Byte Packing4/2(Out2) -> Mux/16
  Dummy/1 -> WFT Byte Packing9/1(In1), WFT Byte Packing4/1(In1), WFT Byte Packing6/1(In1), WFT Byte Packing8/1(In1)
  Dummy6/1 -> Selector6/1
  Dummy2/1 -> WFT Byte Packing7/1(In1), WFT Byte Packing1/1(In1)
  WFT Byte Packing15/2(Out2) -> Mux1/2
  Selector3/1 -> WFT Byte Packing10/1(In1)
  Dummy5/1 -> WFT Byte Packing17/1(In1), WFT Byte Packing11/1(In1)
  Dummy4/1 -> WFT Byte Packing19/1(In1), WFT Byte Packing14/1(In1), WFT Byte Packing16/1(In1), WFT Byte Packing18/1(In1)
  In1/1 -> Bus Selector/1
  Bus Selector/1 -> Selector1/1, Selector3/1  "<Fy>"
  Bus Selector/2 -> Selector2/1, Selector/1  "<Mz>"

== system p1_digital_twin_R2023a/Vehicle Chassis Dynamics/Wheel Model ==
  Wheel Torques : Inport
  Tire Forces : Inport  Port=2
  Bus Selector : BusSelector  OutputSignals=Re,Iw
  Divide : Product  Inputs=*/
  Product : Product
  Subtract : Sum  Inputs=+-
  Wheel Accelerations : Outport
  wires:
  Wheel Torques/1 -> Subtract/1
  Tire Forces/1 -> Product/1
  [Vehicle] -> Bus Selector/1
  Bus Selector/1 -> Product/2  "<Re>"
  Product/1 -> Subtract/2
  Subtract/1 -> Divide/1
  Bus Selector/2 -> Divide/2  "<Iw>"
  Divide/1 -> Wheel Accelerations/1

== system p1_digital_twin_R2023a/Vehicle World Motion/Body Fixed to World Coords ==
  Vx : Inport
  Vy : Inport  Port=2
  r : Inport  Port=3
  Grade : Inport  Port=4
  Discrete-Time Integrator : DiscreteIntegrator  gainval=1  InitialCondition=initialE  SampleTime=-1  ICPrevOutput=DiscIntNeverNeededParam  ICPrevScaledInput=DiscIntNeverNeededParam
  Discrete-Time Integrator1 : DiscreteIntegrator  gainval=1  InitialCondition=initialN  SampleTime=-1  ICPrevOutput=DiscIntNeverNeededParam  ICPrevScaledInput=DiscIntNeverNeededParam
  Discrete-Time Integrator2 : DiscreteIntegrator  gainval=1  InitialCondition=initialH  SampleTime=-1  ICPrevOutput=DiscIntNeverNeededParam  ICPrevScaledInput=DiscIntNeverNeededParam
  Discrete-Time Integrator3 : DiscreteIntegrator  gainval=1  InitialCondition=initialU  SampleTime=-1  ICPrevOutput=DiscIntNeverNeededParam  ICPrevScaledInput=DiscIntNeverNeededParam
  Product{1,4..7} (5 alike) : Product  SaturateOnIntegerOverflow=on  OutDataTypeStr=Inherit: Same as first input
  Sum : Sum  Inputs=+-  SaturateOnIntegerOverflow=on
  Sum1 : Sum  SaturateOnIntegerOverflow=on
  Tan : Trigonometry  Operator=tan
  Trigonometric Function2 : Trigonometry
  Trigonometric Function3 : Trigonometry  Operator=cos
  East : Outport
  North : Outport  Port=2
  Up : Outport  Port=3
  Heading : Outport  Port=4
  Vu : Outport  Port=5
  wires:
  Product4/1 -> Sum1/1
  Product6/1 -> Sum/2
  Product7/1 -> Sum1/2
  Trigonometric Function2/1 -> Product4/2, Product6/2
  Discrete-Time Integrator2/1 -> Heading/1, Trigonometric Function3/1, Trigonometric Function2/1  "PSI"
  Sum1/1 -> Discrete-Time Integrator1/1
  Sum/1 -> Discrete-Time Integrator/1
  Trigonometric Function3/1 -> Product5/2, Product7/2
  Discrete-Time Integrator/1 -> East/1  "East"
  Product5/1 -> Sum/1
  Discrete-Time Integrator1/1 -> North/1  "North"
  Vx/1 -> Product1/1, Product5/1, Product4/1
  r/1 -> Discrete-Time Integrator2/1
  Vy/1 -> Product7/1, Product6/1
  Discrete-Time Integrator3/1 -> Up/1
  Grade/1 -> Tan/1
  Tan/1 -> Product1/2
  Product1/1 -> Vu/1, Discrete-Time Integrator3/1
